simulink model "irep_force_control_m15"  (R2015a)
settings: Solver=ode3  StartTime=0.0  StopTime=inf  FixedStep=dt  RelTol=1e-3
InitFcn:
  | IREP_DEPENDENCY
  | init_omni
  | init_filters
  | init_invivo
  | init_telemanipulation
  | init_parker_xyz
  | init_magnetic_tracker
  | init_loadcell
  | init_scopes
  | init_homing
  | init_force_control
  | init_xpc_invivo_simu
undefined symbols (not defined in the file): ang_vel_scale, B_simu, beta, camera_home_voltage, counter_offset, dt, dt_trakstar, E_Y, encoder_counts, epsilon_robust_inverse, FS_LUT_TAU, FS_LUT_WE, gear_ratio, HomingFineEps, HomingRoughEps, HomingRoughVelocity, I1_primary, I1_secondary, I2_primary, I2_secondary, irep_parameters_left, irep_parameters_right, joystick_filter_coeffs, K_d, K_i, K_naive_inv, K_p, k_right, L1l, L1r, L2l, L2r, L_zeus, left_arm_home_voltage, left_x0_parallelogram, LeftArmHomingDirectionVector, LeftArmHomingIntGain, lin_vel_scale, LOADCELL_BIAS, LOADCELL_GAIN, max_conf_space_speed, N_joystick, N_pots, N_trakstar, OmegaMax, OmegaMin, orientation_epsilon, position_epsilon, pots_filter_coeffs, q_eps_backlash, quadrature_mode, r, right_arm_home_voltage, RightArmHomingDirectionVector, RightArmHomingIntGain, screw_pitch, statics_param, tau_compression_bias, tau_compression_gains, tau_neutral_deadband ... (+16)
libraries: slrtlib x39, simulink x23, xpcobsoletelib x23, xpcconteclib x23, xpcrtudplib x12, xpcmeasurementcomputinglib x6, dspswit3 x2, dspsigops x1
(part 2 of 7)

== system irep_force_control_m15/Joint Level PID Control in mm/Bus Creator ==
  In1 : Inport
  Bus Creator : BusCreator  Inputs=23
  Demux : Demux  Outputs=23
  Out1 : Outport
  wires:
  Demux/1 -> Bus Creator/1  "Righ arm - Overall Translational Movement"
  Demux/2 -> Bus Creator/2  "Right arm - Parallelogram Insert"
  Demux/3 -> Bus Creator/3  "Right arm - Parallelogram Deploy"
  Demux/4 -> Bus Creator/4  "Right arm - Proximal Segment X"
  Demux/5 -> Bus Creator/5  "Right arm - Proximal Segment Y"
  Demux/6 -> Bus Creator/6  "Right arm - Distal Segment X"
  Demux/7 -> Bus Creator/7  "Right arm - Distal Segment Y"
  Demux/8 -> Bus Creator/8  "Right arm - Wrist Joint"
  Demux/9 -> Bus Creator/9  "Right arm - Gripper Joint"
  Demux/10 -> Bus Creator/10  "Left arm - Overall Translational Movement"
  Demux/11 -> Bus Creator/11  "Left arm - Parallelogram Insert"
  Demux/12 -> Bus Creator/12  "Left arm - Parallelogram Deploy"
  Demux/13 -> Bus Creator/13  "Left arm - Proximal Segment X"
  Demux/14 -> Bus Creator/14  "Left arm - Proximal Segment Y"
  Demux/15 -> Bus Creator/15  "Left arm - Distal Segment X"
  Demux/16 -> Bus Creator/16  "Left arm - Distal Segment Y"
  Demux/17 -> Bus Creator/17  "Left arm - Wrist Joint"
  Demux/18 -> Bus Creator/18  "Left arm - Gripper Joint"
  Demux/19 -> Bus Creator/19  "Camera shell open"
  Demux/20 -> Bus Creator/20  "Camera Pan"
  Demux/21 -> Bus Creator/21  "Camera Tilt"
  Bus Creator/1 -> Out1/1
  In1/1 -> Demux/1
  Demux/22 -> Bus Creator/22  "Parker insertion stage"
  Demux/23 -> Bus Creator/23  "Parker rotary stage"

== system irep_force_control_m15/Joint Level PID Control in mm/Bus selector ==
  sensors : Inport
  Camera selector : Subsystem
  Left arm selector : Subsystem
  Mux : Mux
  RZ : Subsystem
  Right arm selector : Subsystem
  Out1 : Outport
  wires:
  Left arm selector/1(Out1) -> Mux/2
  Right arm selector/1(Out1) -> Mux/1
  Camera selector/1(Out1) -> Mux/3
  Mux/1 -> Out1/1
  sensors/1 -> Left arm selector/1(In1), Right arm selector/1(In1), Camera selector/1(In1), RZ/1(In1)
  RZ/1(Out1) -> Mux/4

== system irep_force_control_m15/Joint Level PID Control in mm/PID Compensator ==
  e : Inport
  Enable : EnablePort  StatesWhenEnabling=reset
  Add : Sum  Inputs=+++
  Discrete Derivative : simulink/Discrete/Discrete Derivative  gainval=1.0  ICPrevScaledInput=0.0  InputProcessing=Inherited  OutMin=[]  OutMax=[]  OutDataType=sfix(16)  OutScaling=2^-10  DoSatur=off
  Discrete-Time Integrator : DiscreteIntegrator  SampleTime=dt
  Integral Sat : Saturate  UpperLimit=5  LowerLimit=-5
  Kd : Gain  Gain=K_d  SampleTime=dt
  Ki : Gain  Gain=K_i  SampleTime=dt
  Kp : Gain  Gain=K_p  SampleTime=dt
  Saturation : Saturate  UpperLimit=10  LowerLimit=-10
  u : Outport  InitialOutput=zeros(23,1)
  wires:
  Discrete Derivative/1 -> Add/3
  Kd/1 -> Discrete Derivative/1
  Integral Sat/1 -> Add/2
  Discrete-Time Integrator/1 -> Integral Sat/1
  Saturation/1 -> u/1
  Add/1 -> Saturation/1
  Ki/1 -> Discrete-Time Integrator/1
  Kp/1 -> Add/1
  e/1 -> Ki/1, Kp/1, Kd/1

== system irep_force_control_m15/Scopes/Friction Estimation Data UDP ==
  note: ConfigSpace:
      | b0 [1x1]
      | b1 [2x1]
      | psi [4x1]
      | gamma [1x1]
  note: [9x1]
  note: [4x1]
  note: [6x1]
  note: [6x1]
  note: [6x1]
  note: [6x1]
  sensors : Inport
  ConfigComd : Inport  Port=2
  Clock : Inport  Port=3
  Enable : EnablePort
  Bus Selector1 : BusSelector  OutputSignals=Magnetic Sensors.s1,Magnetic Sensors.s2,Magnetic Sensors.s3,Magnetic Sensors.s4
  Bus Selector2 : BusSelector  OutputSignals=force_sensing.loadcell
  Bus Selector4 : BusSelector  OutputSignals=A/D signals.right arm pots
  Demux : Demux  Outputs=[1 6 1]
  Demux2 : Demux  Outputs=[9 1]
  Mux : Mux  Inputs=10
  Right arm joint def : Subsystem
  STOP : Constant  Value=0
  Terminator{,1..3} (4 alike) : Terminator
  wires:
  sensors/1 -> Right arm joint def/1(sensors), Bus Selector4/1, Bus Selector2/1, Bus Selector1/1
  Bus Selector2/1 -> Mux/3  "<loadcell>"
  Bus Selector1/1 -> Mux/4  "<s1>"
  Bus Selector1/2 -> Mux/5  "<s2>"
  Bus Selector1/3 -> Mux/6  "<s3>"
  Bus Selector1/4 -> Mux/7  "<s4>"
  Right arm joint def/1(right q_cur) -> Mux/1  "q_cur [9x1]"
  ConfigComd/1 -> Demux/1
  Demux/1 -> Terminator/1
  Demux/2 -> Mux/8  "b,psi [6x1]"
  Clock/1 -> Mux/9  "clock [1x1]"
  Mux/1 -> Terminator3/1
  STOP/1 -> Mux/10
  Demux/3 -> Terminator1/1
  Bus Selector4/1 -> Demux2/1  "<right arm pots>"
  Demux2/1 -> Mux/2
  Demux2/2 -> Terminator2/1

== system irep_force_control_m15/Scopes/Left arm joint def ==
  In1 : Inport
  Bus Selector5 : BusSelector  OutputSignals=q.Left arm - overall translational movement,q.Left arm - parallelogram insert joint,q.Left arm - parallelogram deployment joint,q.Left arm - proximal segment - bending in X,q.Left arm - proximal segment - bending in Y,q.Left arm - distal segment - bending in x,q.Left arm - distal segment - bending in y,q.Left arm - wrist,q.Left arm - gripper joint
  Mux5 : Mux  Inputs=9
  Out1 : Outport
  wires:
  Bus Selector5/1 -> Mux5/1  "<Left arm - overall translational movement>"
  Bus Selector5/2 -> Mux5/2  "<Left arm - parallelogram insert joint>"
  Bus Selector5/3 -> Mux5/3  "<Left arm - parallelogram deployment joint>"
  Bus Selector5/4 -> Mux5/4  "<Left arm - proximal segment - bending in X>"
  Bus Selector5/5 -> Mux5/5  "<Left arm - proximal segment - bending in Y>"
  Bus Selector5/6 -> Mux5/6  "<Left arm - distal segment - bending in x>"
  Bus Selector5/7 -> Mux5/7  "<Left arm - distal segment - bending in y>"
  Bus Selector5/8 -> Mux5/8  "<Left arm - wrist>"
  Bus Selector5/9 -> Mux5/9  "<Left arm - gripper joint>"
  In1/1 -> Bus Selector5/1
  Mux5/1 -> Out1/1

== system irep_force_control_m15/Scopes/Magnetic Sensor Scopes ==
  In1 : Inport
  Bus Selector4 : BusSelector  OutputSignals=Magnetic Sensors.s1
  Bus Selector5 : BusSelector  OutputSignals=Magnetic Sensors.s2
  Bus Selector6 : BusSelector  OutputSignals=Magnetic Sensors.s3
  Bus Selector7 : BusSelector  OutputSignals=Magnetic Sensors.s4
  Scope M sensor 1 : slrtlib/Displays and Logging/Scope   scopeno=22  scopetype=Host  autostart=on  viewmode=Numerical  formatstr=scope_format_Msensor_1  grid=on  ylimits=[0,0]  nosamples=50  noprepostsamples=0  interleave=1  triggermode=FreeRun  triggersignal=1  trigsignalfromport=off  triggerlevel=0.0  triggerslope=Either  triggerscope=1  triggersample=0  filename=data.dat  mode=Lazy  writesize=512  autorestart=off  dynamicfilemode=off  maxwritefilesize=512*1024^2
  Scope M sensor 2 : slrtlib/Displays and Logging/Scope   scopeno=23  scopetype=Host  autostart=off  viewmode=Numerical  formatstr=scope_format_Msensor_2  grid=on  ylimits=[0,0]  nosamples=50  noprepostsamples=0  interleave=1  triggermode=FreeRun  triggersignal=1  trigsignalfromport=off  triggerlevel=0.0  triggerslope=Either  triggerscope=1  triggersample=0  filename=data.dat  mode=Lazy  writesize=512  autorestart=off  dynamicfilemode=off  maxwritefilesize=512*1024^2
  "Scope M sensor 3 " : slrtlib/Displays and Logging/Scope   scopeno=30  scopetype=Host  autostart=on  viewmode=Numerical  formatstr=scope_format_Msensor_3  grid=on  ylimits=[0,0]  nosamples=50  noprepostsamples=0  interleave=1  triggermode=FreeRun  triggersignal=1  trigsignalfromport=off  triggerlevel=0.0  triggerslope=Either  triggerscope=1  triggersample=0  filename=data.dat  mode=Lazy  writesize=512  autorestart=off  dynamicfilemode=off  maxwritefilesize=512*1024^2
  Scope M sensor 4 : slrtlib/Displays and Logging/Scope   scopeno=31  scopetype=Host  autostart=on  viewmode=Numerical  formatstr=scope_format_Msensor_4  grid=on  ylimits=[0,0]  nosamples=50  noprepostsamples=0  interleave=1  triggermode=FreeRun  triggersignal=1  trigsignalfromport=off  triggerlevel=0.0  triggerslope=Either  triggerscope=1  triggersample=0  filename=data.dat  mode=Lazy  writesize=512  autorestart=off  dynamicfilemode=off  maxwritefilesize=512*1024^2
  wires:
  Bus Selector4/1 -> Scope M sensor 1/1  "<s1>"
  Bus Selector5/1 -> Scope M sensor 2/1  "<s2>"
  Bus Selector6/1 -> "Scope M sensor 3 "/1  "<s3>"
  Bus Selector7/1 -> Scope M sensor 4/1  "<s4>"
  In1/1 -> Bus Selector6/1, Bus Selector7/1, Bus Selector5/1, Bus Selector4/1

== system irep_force_control_m15/Scopes/Other_scope ==
  In1 : Inport
  Bus Selector2 : BusSelector  OutputSignals=A/D signals.right arm pots,A/D signals.left arm pots,q.Parker insertion stage,q.Parker rotary stage,q.Camera shell open,q.Camera Pan,q.Camera Tilt,foot switches,Pots_Connect
  Camera : slrtlib/Displays and Logging/Scope   scopeno=6  scopetype=Host  autostart=on  viewmode=Numerical  formatstr='Camera: %3.3f'  grid=on  ylimits=[0,0]  nosamples=10  noprepostsamples=0  interleave=1  triggermode=FreeRun  triggersignal=1  trigsignalfromport=off  triggerlevel=0.0  triggerslope=Either  triggerscope=1  triggersample=0  filename=weights1.dat  mode=Lazy  writesize=512  autorestart=off  dynamicfilemode=off  maxwritefilesize=512*1024^2
  Digital Input : slrtlib/Displays and Logging/Scope   scopeno=2  scopetype=Host  autostart=on  viewmode=Numerical  formatstr=scope_format_digital_input  grid=on  ylimits=[0,0]  nosamples=10  noprepostsamples=0  interleave=1  triggermode=FreeRun  triggersignal=1  trigsignalfromport=off  triggerlevel=0.0  triggerslope=Either  triggerscope=1  triggersample=0  filename=weights1.dat  mode=Lazy  writesize=512  autorestart=off  dynamicfilemode=off  maxwritefilesize=512*1024^2
  Left Arm Pots : slrtlib/Displays and Logging/Scope   scopeno=7  scopetype=Target  autostart=on  viewmode=Numerical  formatstr=scope_format_left_pot  grid=on  ylimits=[0,0]  nosamples=10  noprepostsamples=0  interleave=1  triggermode=FreeRun  triggersignal=1  trigsignalfromport=off  triggerlevel=0.0  triggerslope=Either  triggerscope=1  triggersample=0  filename=weights1.dat  mode=Lazy  writesize=512  autorestart=off  dynamicfilemode=off  maxwritefilesize=512*1024^2
  Mux2 : Mux  Inputs=2
  Mux3 : Mux  Inputs=3
  Mux4 : Mux  Inputs=2
  Parker Feedback : slrtlib/Displays and Logging/Scope   scopeno=4  scopetype=Host  autostart=on  viewmode=Numerical  formatstr=scope_format_parker_cur  grid=on  ylimits=[0,0]  nosamples=10  noprepostsamples=0  interleave=1  triggermode=FreeRun  triggersignal=1  trigsignalfromport=off  triggerlevel=0.0  triggerslope=Either  triggerscope=1  triggersample=0  filename=weights1.dat  mode=Lazy  writesize=512  autorestart=off  dynamicfilemode=off  maxwritefilesize=512*1024^2
  Right Arm Pots : slrtlib/Displays and Logging/Scope   scopeno=8  scopetype=Target  autostart=on  viewmode=Numerical  formatstr=scope_format_right_pot  grid=on  ylimits=[0,0]  nosamples=10  noprepostsamples=0  interleave=1  triggermode=FreeRun  triggersignal=1  trigsignalfromport=off  triggerlevel=0.0  triggerslope=Either  triggerscope=1  triggersample=0  filename=weights1.dat  mode=Lazy  writesize=512  autorestart=off  dynamicfilemode=off  maxwritefilesize=512*1024^2
  wires:
  Bus Selector2/1 -> Right Arm Pots/1  "<right arm pots>"
  Bus Selector2/2 -> Left Arm Pots/1  "<left arm pots>"
  Bus Selector2/3 -> Mux2/1  "<Parker insertion stage>"
  Bus Selector2/4 -> Mux2/2  "<Parker rotary stage>"
  Mux2/1 -> Parker Feedback/1
  Mux3/1 -> Camera/1
  Bus Selector2/5 -> Mux3/1  "<Camera shell open>"
  Bus Selector2/6 -> Mux3/2  "<Camera Pan>"
  Bus Selector2/7 -> Mux3/3  "<Camera Tilt>"
  Bus Selector2/8 -> Mux4/1  "<foot switches>"
  Bus Selector2/9 -> Mux4/2  "<Pots_Connect>"
  Mux4/1 -> Digital Input/1
  In1/1 -> Bus Selector2/1

== system irep_force_control_m15/Scopes/Right arm joint def ==
  In1 : Inport
  Bus Selector4 : BusSelector  OutputSignals=q.Right arm - overall translational movement,q.Right arm - parallelogram insert joint,q.Right arm - parallelogram deployment joint,q.Right arm - Proximal segment - bending in X,q.Righ arm - Proximal segment - bending in Y,q.Right arm - distal segment - bending in X,q.Right arm - distal segment - bending in Y,q.Right arm - wrist,q.Right arm - Gripper Joint
  Mux1 : Mux  Inputs=9
  Out1 : Outport
  wires:
  Bus Selector4/1 -> Mux1/1  "<Right arm - overall translational movement>"
  Bus Selector4/2 -> Mux1/2  "<Right arm - parallelogram insert joint>"
  Bus Selector4/3 -> Mux1/3  "<Right arm - parallelogram deployment joint>"
  Bus Selector4/4 -> Mux1/4  "<Right arm - Proximal segment - bending in X>"
  Bus Selector4/5 -> Mux1/5  "<Righ arm - Proximal segment - bending in Y>"
  Bus Selector4/6 -> Mux1/6  "<Right arm - distal segment - bending in X>"
  Bus Selector4/7 -> Mux1/7  "<Right arm - distal segment - bending in Y>"
  Bus Selector4/8 -> Mux1/8  "<Right arm - wrist>"
  Bus Selector4/9 -> Mux1/9  "<Right arm - Gripper Joint>"
  In1/1 -> Bus Selector4/1
  Mux1/1 -> Out1/1

== system irep_force_control_m15/Scopes/left ==
  In1 : Inport
  Bus Selector : BusSelector  OutputSignals=Left arm - Proximal Segment Y,Left arm - Gripper Joint,Left arm - Proximal Segment X,Left arm - Distal Segment X,Left arm - Wrist Joint,Left arm - Distal Segment Y,Left arm - Parallelogram Deploy,Left arm - Parallelogram Insert,Left arm - Overall Translational Movement
  Gain{1..4} (4 alike) : Gain  Gain=-1
  Mux : Mux  Inputs=9
  Out1 : Outport
  wires:
  Bus Selector/1 -> Gain1/1  "<Left arm - Proximal Segment Y>"
  Bus Selector/2 -> Mux/2  "<Left arm - Gripper Joint>"
  Bus Selector/4 -> Mux/4  "<Left arm - Distal Segment X>"
  Bus Selector/5 -> Mux/5  "<Left arm - Wrist Joint>"
  Bus Selector/6 -> Gain2/1  "<Left arm - Distal Segment Y>"
  Bus Selector/7 -> Gain3/1  "<Left arm - Parallelogram Deploy>"
  Bus Selector/8 -> Gain4/1  "<Left arm - Parallelogram Insert>"
  In1/1 -> Bus Selector/1
  Mux/1 -> Out1/1
  Bus Selector/3 -> Mux/3  "<Left arm - Proximal Segment X>"
  Gain1/1 -> Mux/1
  Gain2/1 -> Mux/6
  Gain3/1 -> Mux/7
  Gain4/1 -> Mux/8
  Bus Selector/9 -> Mux/9  "<Left arm - Overall Translational Movement>"

== system irep_force_control_m15/Scopes/parker ==
  In1 : Inport
  Bus Selector : BusSelector  OutputSignals=Parker insertion stage,Parker rotary stage
  Gain1 : Gain  Gain=-1
  Gain2 : Gain  Gain=-1
  Mux : Mux  Inputs=2
  Out1 : Outport
  wires:
  Bus Selector/1 -> Gain1/1  "<Parker insertion stage>"
  Bus Selector/2 -> Gain2/1  "<Parker rotary stage>"
  In1/1 -> Bus Selector/1
  Mux/1 -> Out1/1
  Gain1/1 -> Mux/1
  Gain2/1 -> Mux/2

== system irep_force_control_m15/Scopes/right ==
  In1 : Inport
  Bus Selector : BusSelector  OutputSignals=Right arm - Proximal Segment Y,Right arm - Gripper Joint,Right arm - Proximal Segment X,Right arm - Distal Segment X,Right arm - Wrist Joint,Right arm - Distal Segment Y,Right arm - Parallelogram Deploy,Right arm - Parallelogram Insert,Righ arm - Overall Translational Movement
  Mux : Mux  Inputs=9
  Out1 : Outport
  wires:
  In1/1 -> Bus Selector/1
  Mux/1 -> Out1/1
  Bus Selector/3 -> Mux/3  "<Right arm - Proximal Segment X>"
  Bus Selector/4 -> Mux/4  "<Right arm - Distal Segment X>"
  Bus Selector/5 -> Mux/5  "<Right arm - Wrist Joint>"
  Bus Selector/6 -> Mux/6  "<Right arm - Distal Segment Y>"
  Bus Selector/8 -> Mux/8  "<Right arm - Parallelogram Insert>"
  Bus Selector/2 -> Mux/2  "<Right arm - Gripper Joint>"
  Bus Selector/1 -> Mux/1  "<Right arm - Proximal Segment Y>"
  Bus Selector/7 -> Mux/7  "<Right arm - Parallelogram Deploy>"
  Bus Selector/9 -> Mux/9  "<Righ arm - Overall Translational Movement>"

== system irep_force_control_m15/Scopes/select force ==
  wrench est : Inport
  Bus Selector4 : BusSelector  OutputSignals=Ws_right,Ws_uncomp,We_right_seg1,Ws_bias
  Demux{,1..3} (4 alike) : Demux  Outputs=[3,3]
  Mux : Mux  Inputs=3
  Terminator{,1..4} (5 alike) : Terminator
  Force : Outport
  wires:
  Bus Selector4/1 -> Demux/1  "<Ws_right>"
  Bus Selector4/3 -> Demux1/1  "<We_right_seg1>"
  Demux/2 -> Terminator/1  "Torque"
  Demux1/2 -> Terminator1/1  "Torque"
  Demux/1 -> Mux/1  "Force"
  Mux/1 -> Force/1
  wrench est/1 -> Bus Selector4/1
  Demux1/1 -> Terminator2/1  "Force"
  Bus Selector4/2 -> Demux2/1  "<Ws_uncomp>"
  Demux2/2 -> Terminator3/1
  Demux2/1 -> Mux/2
  Bus Selector4/4 -> Demux3/1  "<Ws_bias>"
  Demux3/2 -> Terminator4/1
  Demux3/1 -> Mux/3

== system irep_force_control_m15/Trajectory Planner/Camera ==
  vision : Inport
  sensors : Inport  Port=2
  Enable : EnablePort
  Enable Homing : Constant  Value=0  SampleTime=dt
  Enable Joint Space : Constant  Value=0  SampleTime=dt
  Enable Joystick : Constant  Value=0  SampleTime=dt
  Enable Tool Tracking : Constant  Value=0  SampleTime=dt
  Homing Procedure : Subsystem  TreatAsAtomicUnit=on
  Joint Space : Subsystem  TreatAsAtomicUnit=on
  Joystick Control for Cam : Subsystem  TreatAsAtomicUnit=on
  Merge : Merge  Inputs=4  InitialOutput=zeros(3,1)
  Saturation : Saturate  UpperLimit=[5 1.6 1.5]  LowerLimit=[-5 -1.6 -1.5]
  Tool Tracking : Subsystem  TreatAsAtomicUnit=on
  q des camera : Outport  InitialOutput=zeros(3,1)
  wires:
  Enable Tool Tracking/1 -> Tool Tracking/Enable
  Merge/1 -> Saturation/1
  vision/1 -> Tool Tracking/1(tool XY)
  Enable Joint Space/1 -> Joint Space/Enable
  sensors/1 -> Joystick Control for Cam/1(sensors), Homing Procedure/1(sensors)
  Enable Joystick/1 -> Joystick Control for Cam/Enable
  Homing Procedure/1(q des) -> Merge/1
  Joint Space/1(Out1) -> Merge/2
  Tool Tracking/1(q des) -> Merge/3
  Joystick Control for Cam/1(q des) -> Merge/4
  Enable Homing/1 -> Homing Procedure/Enable
  Saturation/1 -> q des camera/1

== system irep_force_control_m15/Trajectory Planner/Delay_test ==
  Delay_test : xpcrtudplib/Legacy UDP/Send   ipAddress=192.168.1.64  ipPort=10031  localPort=-1  vblLen=off  sampletime=0.01
  Digital Clock : DigitalClock  SampleTime=dt
  Pack1 : xpcobsoletelib/Utilities/Pack   datatypes={'double'}  byteAlign=1
  Receive : xpcrtudplib/Legacy UDP/Receive   ipAddress=0.0.0.0  ipPort=10030  width=8  vblLen=on  sampletime=0.01
  "Scope (xPC) " : slrtlib/Displays and Logging/Scope   scopeno=25  scopetype=Host  autostart=on  viewmode=Numerical  formatstr='Delay:%15.6f'  grid=on  ylimits=[0,0]  nosamples=250  noprepostsamples=0  interleave=1  triggermode=FreeRun  triggersignal=1  trigsignalfromport=off  triggerlevel=0.0  triggerslope=Either  triggerscope=1  triggersample=0  filename=data.dat  mode=Lazy  writesize=512  autorestart=off  dynamicfilemode=off  maxwritefilesize=512*1024^2
  Sum : Sum  Inputs=|+-
  Terminator : Terminator
  Unpack : xpcobsoletelib/Utilities/Unpack   dimensions={1}  datatypes={'double'}  byteAlign=1
  wires:
  Digital Clock/1 -> Pack1/1, Sum/1
  Pack1/1 -> Delay_test/1
  Receive/2 -> Terminator/1
  Receive/1 -> Unpack/1
  Unpack/1 -> Sum/2
  Sum/1 -> "Scope (xPC) "/1

== system irep_force_control_m15/Trajectory Planner/Left Arm ==
  note: IREP Left Arm Trajectory Planner - v 0.6 - © COPYRIGHT 2011 Andrea Bajo, Nabil Simaan
  Master : Inport
  sensors : Inport  Port=2
  Enable : EnablePort
  Enable High Level : Constant  Value=0  SampleTime=dt
  Enable Low Level : Constant  Value=0  SampleTime=dt
  High Level : Subsystem  TreatAsAtomicUnit=on
  Low Level : Subsystem  TreatAsAtomicUnit=on
  Merge1 : Merge  InitialOutput=zeros(9,1)
  q left arm : Outport  InitialOutput=zeros(9,1)
  conf space : Outport  Port=2
  b0 dot left : Outport  Port=3
  TASK_EN : Outport  Port=4
  current_pose : Outport  Port=5
  wires:
  Enable Low Level/1 -> Low Level/Enable
  Low Level/1(q des) -> Merge1/1
  Enable High Level/1 -> High Level/Enable
  High Level/1(q des) -> Merge1/2
  sensors/1 -> Low Level/1(sensors), High Level/2(sensors)
  Master/1 -> High Level/1(Master)
  Merge1/1 -> q left arm/1
  High Level/2(conf space) -> conf space/1
  High Level/3(b0_dot_left) -> b0 dot left/1
  High Level/4(TASK_EN) -> TASK_EN/1
  High Level/5(current_pose) -> current_pose/1

== system irep_force_control_m15/Trajectory Planner/RZ ==
  trajectory : Inport
  sensors : Inport  Port=2
  Enable : EnablePort
  Add : Sum
  Arm selector : MATLAB Function  TreatAsAtomicUnit=on
  Bus Selector1 : BusSelector  OutputSignals=right arm.b0 dot right,left arm.b0 dot left
  Discrete-Time Integrator : DiscreteIntegrator  InitialCondition=[0;0]  SampleTime=dt  LimitOutput=on  UpperSaturationLimit=[200;pi/2]  LowerSaturationLimit=[-100;0]
  Enable Joint Space : Constant  Value=0  SampleTime=dt
  Joystick Control for RZ : Subsystem  TreatAsAtomicUnit=on
  Subsystem : Subsystem
  Parker : Outport  InitialOutput=zeros(2,1)
  wires:
  sensors/1 -> Joystick Control for RZ/1(sensors)
  Joystick Control for RZ/1(q des) -> Subsystem/1(In1)
  Enable Joint Space/1 -> Joystick Control for RZ/Enable
  Add/1 -> Discrete-Time Integrator/1
  Subsystem/1(Out1) -> Add/2
  Arm selector/1(b0dot) -> Add/1
  Discrete-Time Integrator/1 -> Parker/1
  trajectory/1 -> Bus Selector1/1
  Bus Selector1/1 -> Arm selector/1(right_b0_dot)  "<b0 dot right>"
  Bus Selector1/2 -> Arm selector/2(left_b0_dot)  "<b0 dot left>"

== system irep_force_control_m15/Trajectory Planner/Right Arm ==
  note: IREP Right Arm Trajectory Planner - v 1.0 - © COPYRIGHT 2011 Andrea Bajo, Nabil Simaan
  Master : Inport
  sensors : Inport  Port=2
  Enable : EnablePort
  Enable High Level : Constant  Value=0  SampleTime=dt
  Enable Low Level : Constant  Value=0  SampleTime=dt
  High Level : Subsystem  TreatAsAtomicUnit=on
  Low Level : Subsystem  TreatAsAtomicUnit=on
  Merge1 : Merge  InitialOutput=zeros(9,1)
  conf space : Outport  PortDimensions=8
  q right arm : Outport  Port=2  InitialOutput=zeros(9,1)
  b0 dot right : Outport  Port=3
  TASK_EN : Outport  Port=4
  current_pose : Outport  Port=5
  q dot sgn : Outport  Port=6
  wires:
  Enable Low Level/1 -> Low Level/Enable
  Low Level/1(q des) -> Merge1/1
  Enable High Level/1 -> High Level/Enable
  High Level/1(q des) -> Merge1/2
  sensors/1 -> Low Level/1(sensors), High Level/2(sensors)
  Master/1 -> High Level/1(Master)
  High Level/2(conf space) -> conf space/1
  High Level/3(b0 dot) -> b0 dot right/1
  High Level/4(TASK_EN) -> TASK_EN/1
  Merge1/1 -> q right arm/1
  High Level/5(current_pose) -> current_pose/1
  High Level/6(q dot sgn) -> q dot sgn/1

== system irep_force_control_m15/Trajectory Planner/Signals packing ==
  irep : Inport
  parker : Inport  Port=2
  Bus Creator : BusCreator
  Bus Selector : BusSelector  OutputSignals=right arm.q des right,left arm.q des left,camera q
  system : Outport
  wires:
  Bus Selector/1 -> Bus Creator/1  "<q des right>"
  Bus Selector/2 -> Bus Creator/2  "<q des left>"
  Bus Selector/3 -> Bus Creator/3  "<camera q>"
  irep/1 -> Bus Selector/1
  Bus Creator/1 -> system/1
  parker/1 -> Bus Creator/4

== system irep_force_control_m15/Trajectory Planner/UDP_SendTo_MTM ==
  Traj : Inport
  Right_MTM : Inport  Port=2
  Left_MTM : Inport  Port=3
  Right_Wrench : Inport  Port=4
  Left_UDP : Subsystem
  Right_UDP : Subsystem
  wires:
  Traj/1 -> Right_UDP/1(traj), Left_UDP/1(traj)
  Right_MTM/1 -> Right_UDP/2(MTM)
  Left_MTM/1 -> Left_UDP/2(MTM)
  Right_Wrench/1 -> Right_UDP/3(Wrench)

== system irep_force_control_m15/Wrench Estimation/Wrench Compensation ==
  note: Compensation Mode
  note: Compensation using lookup tables
  Ws : Inport
  q_dot_sign : Inport  Port=2
  psi : Inport  Port=3
  Compare To Constant1 : simulink/Logic and Bit Operations/Compare To Constant  relop===  const=1  OutDataTypeStr=boolean
  Constant : Constant  Value=zeros(12,1)
  Multiport Switch : MultiPortSwitch  DataPortOrder=Specify indices  DataPortIndices={1,0}
  Sum : Sum  Inputs=+-|
  wrench comp mode : Constant  Value=0
  wrench sensing compensation LUT : Subsystem
  Ws_comp : Outport
  Ws_bias : Outport  Port=2
  wires:
  [mode] -> Multiport Switch/1
  wrench comp mode/1 -> [mode]
  Multiport Switch/1 -> Ws_bias/1, Sum/2
  [mode] -> Compare To Constant1/1
  Compare To Constant1/1 -> wrench sensing compensation LUT/Enable
  q_dot_sign/1 -> wrench sensing compensation LUT/1(q_dot_sign)
  psi/1 -> wrench sensing compensation LUT/2(psi)
  wrench sensing compensation LUT/1(ws_bias) -> Multiport Switch/2
  Ws/1 -> Sum/1
  Sum/1 -> Ws_comp/1
  Constant/1 -> Multiport Switch/3

== system irep_force_control_m15/Wrench Estimation/Wrench Est Right Arm ==
  note: Ws - the estimated wrench at the tip of the robot
      | We_seg1 - the estimated wrench at the end of the 1st segment
      | tau_comp - the compensated tau
  tau : Inport
  psi : Inport  Port=2
  Constant : Constant  Value=r
  Constant1 : Constant  Value=[1 0 0]
  Constant2 : Constant  Value=[0 1 0]
  Constant3 : Constant
  Constant4 : Constant
  Constant5 : Constant  Value=0
  Mux : Mux  Inputs=2
  Sample and Hold : dspsigops/Sample and Hold  trig=Rising edge  initCond=0  latchinput=off
  Sum : Sum  Inputs=|+-
  compute wrench est : MATLAB Function  TreatAsAtomicUnit=on
  reset : Constant  Value=0
  robot kin param : Constant  Value=irep_parameters_right
  robot statics param : Constant  Value=statics_param
  sel param : Subsystem
  Ws : Outport
  wires:
  Constant/1 -> compute wrench est/8(r)
  Constant1/1 -> compute wrench est/3(n_t)
  Constant2/1 -> compute wrench est/4(n_n)
  Constant3/1 -> compute wrench est/5(c_t)
  Constant4/1 -> compute wrench est/6(c_n)
  robot kin param/1 -> sel param/1(In)
  sel param/1(L) -> compute wrench est/7(L)
  robot statics param/1 -> compute wrench est/9(statics_param)
  Constant5/1 -> compute wrench est/10(probe_offset)
  psi/1 -> compute wrench est/2(Psi)
  tau/1 -> compute wrench est/1(tau_curr)
  reset/1 -> Sample and Hold/Trigger
  Mux/1 -> Sum/1, Sample and Hold/1
  Sample and Hold/1 -> Sum/2
  compute wrench est/1(Ws) -> Mux/1
  compute wrench est/2(W_seg1) -> Mux/2
  Sum/1 -> Ws/1

== system irep_force_control_m15/Wrench Estimation/combine psi ==
  note: Combining measured psi and commanded psi
      | measured psi has a good estimate of theta
      | but very poor estimate of delta
  psi_d : Inport
  psi_m : Inport  Port=2
  Demux : Demux  Outputs=[4,1]
  Sum : Sum  Inputs=|++
  Terminator : Terminator
  select desired : Gain  Gain=[1,1,1,1]
  select measured : Gain  Gain=[0,0,0,0]
  psi : Outport
  wires:
  psi_m/1 -> select measured/1
  Sum/1 -> psi/1
  Demux/2 -> Terminator/1
  Demux/1 -> select desired/1
  select measured/1 -> Sum/1
  select desired/1 -> Sum/2
  psi_d/1 -> Demux/1

== system irep_force_control_m15/Wrench Estimation/q_cur to q_bb ==
  q_cur : Inport
  Bus Selector1 : BusSelector  OutputSignals=q.Right arm - Proximal segment - bending in X,q.Righ arm - Proximal segment - bending in Y,q.Right arm - distal segment - bending in X,q.Right arm - distal segment - bending in Y
  Gain{,1..3} (4 alike) : Gain  Gain=-1
  Mux1 : Mux  Inputs=8
  q_bb : Outport
  wires:
  q_cur/1 -> Bus Selector1/1
  Mux1/1 -> q_bb/1
  Bus Selector1/1 -> Mux1/1, Gain/1  "<Right arm - Proximal segment - bending in X>"
  Bus Selector1/2 -> Mux1/2, Gain1/1  "<Righ arm - Proximal segment - bending in Y>"
  Bus Selector1/3 -> Mux1/5, Gain2/1  "<Right arm - distal segment - bending in X>"
  Bus Selector1/4 -> Mux1/6, Gain3/1  "<Right arm - distal segment - bending in Y>"
  Gain/1 -> Mux1/3
  Gain1/1 -> Mux1/4
  Gain2/1 -> Mux1/7
  Gain3/1 -> Mux1/8

== system irep_force_control_m15/Wrench Estimation/signal packing ==
  note: Ws_right - the estimated wrench at the tip of the robot
      | We_right_seg1 - the estimated wrench at the end of the 1st segment
      | tau_comp - the compensated tau
  tau_comp : Inport
  Ws : Inport  Port=2
  Ws_uncomp : Inport  Port=3
  Ws_bias : Inport  Port=4
  Bus Creator : BusCreator  Inputs=5
  Demux : Demux  Outputs=[6,6]
  Demux1 : Demux  Outputs=[6,6]
  Demux2 : Demux  Outputs=[6,6]
  Terminator : Terminator
  Terminator1 : Terminator
  wrench_est : Outport
  wires:
  Ws/1 -> Demux/1
  Demux/1 -> Bus Creator/2  "Ws_right"
  tau_comp/1 -> Bus Creator/1  "tau_comp"
  Demux/2 -> Bus Creator/3  "We_right_seg1"
  Bus Creator/1 -> wrench_est/1  "wrench_est"
  Ws_uncomp/1 -> Demux1/1
  Demux1/2 -> Terminator/1
  Demux1/1 -> Bus Creator/4  "Ws_uncomp"
  Ws_bias/1 -> Demux2/1
  Demux2/2 -> Terminator1/1
  Demux2/1 -> Bus Creator/5  "Ws_bias"

== system irep_force_control_m15/Wrench Estimation/tau sensing compensation ==
  note: Compensation using gain model
  note: Compensation using lookup tables
  note: Compensation Mode
  q_bb : Inport
  tau_measured : Inport  Port=2
  q_dot_sign : Inport  Port=3
  psi : Inport  Port=4
  Compare To Constant : simulink/Logic and Bit Operations/Compare To Constant  relop===  const=1  OutDataTypeStr=boolean
  Compare To Constant1 : simulink/Logic and Bit Operations/Compare To Constant  relop===  const=2  OutDataTypeStr=boolean
  Multiport Switch : MultiPortSwitch  DataPortOrder=Specify indices  DataPortIndices={1,2,0}
  tau comp mode : Constant  Value=0
  tau sensing compensation LUT : Subsystem
  tau sensing compensation gain model : Subsystem
  tau_comp : Outport
  wires:
  tau_measured/1 -> tau sensing compensation LUT/1(tau_measured), Multiport Switch/4, tau sensing compensation gain model/2(tau_sensed)
  q_bb/1 -> tau sensing compensation gain model/1(q_bb)
  tau comp mode/1 -> [mode]
  [mode] -> Compare To Constant/1
  Compare To Constant/1 -> tau sensing compensation gain model/Enable
  [mode] -> Compare To Constant1/1
  Compare To Constant1/1 -> tau sensing compensation LUT/Enable
  q_dot_sign/1 -> tau sensing compensation LUT/2(q_dot_sign)
  psi/1 -> tau sensing compensation LUT/3(psi)
  Multiport Switch/1 -> tau_comp/1
  tau sensing compensation gain model/1(tau_comp) -> Multiport Switch/2
  tau sensing compensation LUT/1(tau_comp) -> Multiport Switch/3
  [mode] -> Multiport Switch/1

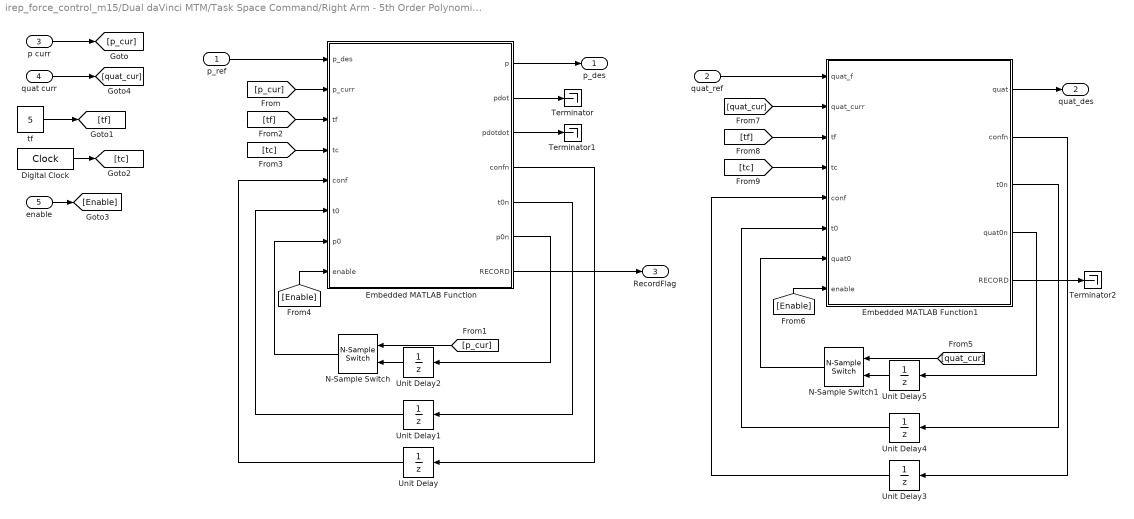
== system irep_force_control_m15/Dual daVinci MTM/Task Space Command/Right Arm - 5th Order Polynomial and Slerp ==
  p_ref : Inport
  quat_ref : Inport  Port=2
  p curr : Inport  Port=3
  quat curr : Inport  Port=4
  enable : Inport  Port=5
  Digital Clock : DigitalClock  SampleTime=dt
  Embedded MATLAB Function : MATLAB Function  TreatAsAtomicUnit=on
  Embedded MATLAB Function1 : MATLAB Function  TreatAsAtomicUnit=on
  N-Sample Switch : dspswit3/N-Sample Switch  N=1  reset=off  TriggerType=Rising edge  Ts=dt
  N-Sample Switch1 : dspswit3/N-Sample Switch  N=1  reset=off  TriggerType=Rising edge  Ts=dt
  Terminator : Terminator
  Terminator1 : Terminator
  Terminator2 : Terminator
  Unit Delay{,1..4} (5 alike) : UnitDelay  SampleTime=dt
  Unit Delay5 : UnitDelay  InitialCondition=[1;0;0;0]  SampleTime=dt
  tf : Constant  Value=5  SampleTime=dt
  p_des : Outport
  quat_des : Outport  Port=2
  RecordFlag : Outport  Port=3
  wires:
  Embedded MATLAB Function/4(confn) -> Unit Delay/1
  Unit Delay/1 -> Embedded MATLAB Function/5(conf)
  Embedded MATLAB Function/5(t0n) -> Unit Delay1/1
  Embedded MATLAB Function/6(p0n) -> Unit Delay2/1
  Unit Delay1/1 -> Embedded MATLAB Function/6(t0)
  p_ref/1 -> Embedded MATLAB Function/1(p_des)
  Embedded MATLAB Function/2(pdot) -> Terminator/1
  Embedded MATLAB Function/3(pdotdot) -> Terminator1/1
  N-Sample Switch/1 -> Embedded MATLAB Function/7(p0)
  Unit Delay2/1 -> N-Sample Switch/2
  p curr/1 -> [p_cur]
  [p_cur] -> Embedded MATLAB Function/2(p_curr)
  [p_cur] -> N-Sample Switch/1
  Embedded MATLAB Function/7(RECORD) -> RecordFlag/1
  Embedded MATLAB Function/1(p) -> p_des/1
  tf/1 -> [tf]
  Digital Clock/1 -> [tc]
  [tf] -> Embedded MATLAB Function/3(tf)
  [tc] -> Embedded MATLAB Function/4(tc)
  enable/1 -> [Enable]
  [Enable] -> Embedded MATLAB Function/8(enable)
  quat_ref/1 -> Embedded MATLAB Function1/1(quat_f)
  quat curr/1 -> [quat_cur]
  Embedded MATLAB Function1/3(t0n) -> Unit Delay4/1
  Embedded MATLAB Function1/4(quat0n) -> Unit Delay5/1
  Unit Delay4/1 -> Embedded MATLAB Function1/6(t0)
  N-Sample Switch1/1 -> Embedded MATLAB Function1/7(quat0)
  Unit Delay5/1 -> N-Sample Switch1/2
  [quat_cur] -> N-Sample Switch1/1
  Embedded MATLAB Function1/2(confn) -> Unit Delay3/1
  Unit Delay3/1 -> Embedded MATLAB Function1/5(conf)
  [Enable] -> Embedded MATLAB Function1/8(enable)
  [quat_cur] -> Embedded MATLAB Function1/2(quat_curr)
  [tf] -> Embedded MATLAB Function1/3(tf)
  [tc] -> Embedded MATLAB Function1/4(tc)
  Embedded MATLAB Function1/1(quat) -> quat_des/1
  Embedded MATLAB Function1/5(RECORD) -> Terminator2/1

== system irep_force_control_m15/Dual daVinci MTM/scopes/to file ==
  right : Inport
  left : Inport  Port=2
  Enable : EnablePort
  Joint Space Info File : slrtlib/Displays and Logging/Scope   scopeno=24  scopetype=File  autostart=on  viewmode=Numerical  formatstr="'tau: %8.3f,     %8.3f,     %8.3f,     %8.3f,     %8.3f,     %8.3f'"  grid=on  ylimits=[0,0]  nosamples=100000  noprepostsamples=0  interleave=1  triggermode=FreeRun  triggersignal=1  trigsignalfromport=off  triggerlevel=0.0  triggerslope=Either  triggerscope=1  triggersample=0  filename=MTMR.dat  mode=Lazy  writesize=512  autorestart=off  dynamicfilemode=off  maxwritefilesize=512*1024^2
  Terminator : Terminator
  wires:
  right/1 -> Joint Space Info File/1
  left/1 -> Terminator/1

== system irep_force_control_m15/In-Vivo System/CONTEC CARDS/Level 1 ==
  note: Contec
      | CNT32-8M (PCI)
      | Inc. Encoder
      | Slot: [1, 13]
  Mux : Mux  Inputs=8
  enc 1 : xpcconteclib/Incremental Encoder/CNT32-8M(PCI)   Channel=1  OperationMode=2-phase Input Synchronous Clear Multiply by 4  DigitalFilter=No filtering  PulseInput=TTL level input  Direction=Up in the clockwise direction/Down in the counterclockwise direction  InitialValue=counter_offset_init  LoadInitialValue=on  SampleTime=dt  PciSlot=[1,13]  StartMethod=Model Start  StopMethod=Model Terminate  ZeroClearRising=off  ZeroClearFalling=off  ZeroClearMatch0=off  ZeroClearMatch1=off  PresetRising=on  PresetFalling=off  PresetMatch0=off  PresetMatch1=off  PresetValue=0  Match0Value=0  Match1Value=0  OutputSignalMatch0=off  OutputSignalMatch1=off  OutputSignalAbnormal=off  OutputSignalDigitalFilter=off  OutputSignalAlarm=off  OneShotDuration=10 microseconds  IndexEnable=Disable  IndexLogic=Positive (Active High)  EnableDigitalInput=off  EnableDigitalOutput=off  DigitalOutputInitialValue=None  DigitalOutputFinalValue=None
  enc 2 : xpcconteclib/Incremental Encoder/CNT32-8M(PCI)   Channel=2  OperationMode=2-phase Input Synchronous Clear Multiply by 4  DigitalFilter=No filtering  PulseInput=TTL level input  Direction=Up in the clockwise direction/Down in the counterclockwise direction  InitialValue=counter_offset_init  LoadInitialValue=on  SampleTime=dt  PciSlot=[1,13]  StartMethod=Model Start  StopMethod=Model Terminate  ZeroClearRising=off  ZeroClearFalling=off  ZeroClearMatch0=off  ZeroClearMatch1=off  PresetRising=off  PresetFalling=off  PresetMatch0=off  PresetMatch1=off  PresetValue=0  Match0Value=0  Match1Value=0  OutputSignalMatch0=off  OutputSignalMatch1=off  OutputSignalAbnormal=off  OutputSignalDigitalFilter=off  OutputSignalAlarm=off  OneShotDuration=10 microseconds  IndexEnable=Disable  IndexLogic=Positive (Active High)  EnableDigitalInput=off  EnableDigitalOutput=off  DigitalOutputInitialValue=None  DigitalOutputFinalValue=None
  enc 3 : xpcconteclib/Incremental Encoder/CNT32-8M(PCI)   Channel=3  OperationMode=2-phase Input Synchronous Clear Multiply by 4  DigitalFilter=No filtering  PulseInput=TTL level input  Direction=Down in the clockwise direction/Up in the counterclockwise direction  InitialValue=counter_offset_init  LoadInitialValue=on  SampleTime=dt  PciSlot=[1,13]  StartMethod=Model Start  StopMethod=Model Terminate  ZeroClearRising=off  ZeroClearFalling=off  ZeroClearMatch0=off  ZeroClearMatch1=off  PresetRising=off  PresetFalling=off  PresetMatch0=off  PresetMatch1=off  PresetValue=0  Match0Value=0  Match1Value=0  OutputSignalMatch0=off  OutputSignalMatch1=off  OutputSignalAbnormal=off  OutputSignalDigitalFilter=off  OutputSignalAlarm=off  OneShotDuration=10 microseconds  IndexEnable=Disable  IndexLogic=Positive (Active High)  EnableDigitalInput=off  EnableDigitalOutput=off  DigitalOutputInitialValue=None  DigitalOutputFinalValue=None
  enc 4 : xpcconteclib/Incremental Encoder/CNT32-8M(PCI)   Channel=4  OperationMode=2-phase Input Synchronous Clear Multiply by 4  DigitalFilter=No filtering  PulseInput=TTL level input  Direction=Down in the clockwise direction/Up in the counterclockwise direction  InitialValue=counter_offset_init  LoadInitialValue=on  SampleTime=dt  PciSlot=[1,13]  StartMethod=Model Start  StopMethod=Model Terminate  ZeroClearRising=off  ZeroClearFalling=off  ZeroClearMatch0=off  ZeroClearMatch1=off  PresetRising=off  PresetFalling=off  PresetMatch0=off  PresetMatch1=off  PresetValue=0  Match0Value=0  Match1Value=0  OutputSignalMatch0=off  OutputSignalMatch1=off  OutputSignalAbnormal=off  OutputSignalDigitalFilter=off  OutputSignalAlarm=off  OneShotDuration=10 microseconds  IndexEnable=Disable  IndexLogic=Positive (Active High)  EnableDigitalInput=off  EnableDigitalOutput=off  DigitalOutputInitialValue=None  DigitalOutputFinalValue=None
  enc 5 : xpcconteclib/Incremental Encoder/CNT32-8M(PCI)   Channel=5  OperationMode=2-phase Input Synchronous Clear Multiply by 4  DigitalFilter=No filtering  PulseInput=TTL level input  Direction=Up in the clockwise direction/Down in the counterclockwise direction  InitialValue=counter_offset_init  LoadInitialValue=on  SampleTime=dt  PciSlot=[1,13]  StartMethod=Model Start  StopMethod=Model Terminate  ZeroClearRising=off  ZeroClearFalling=off  ZeroClearMatch0=off  ZeroClearMatch1=off  PresetRising=off  PresetFalling=off  PresetMatch0=off  PresetMatch1=off  PresetValue=0  Match0Value=0  Match1Value=0  OutputSignalMatch0=off  OutputSignalMatch1=off  OutputSignalAbnormal=off  OutputSignalDigitalFilter=off  OutputSignalAlarm=off  OneShotDuration=10 microseconds  IndexEnable=Disable  IndexLogic=Positive (Active High)  EnableDigitalInput=off  EnableDigitalOutput=off  DigitalOutputInitialValue=None  DigitalOutputFinalValue=None
  enc 6 : xpcconteclib/Incremental Encoder/CNT32-8M(PCI)   Channel=6  OperationMode=2-phase Input Synchronous Clear Multiply by 4  DigitalFilter=No filtering  PulseInput=TTL level input  Direction=Up in the clockwise direction/Down in the counterclockwise direction  InitialValue=counter_offset_init  LoadInitialValue=on  SampleTime=dt  PciSlot=[1,13]  StartMethod=Model Start  StopMethod=Model Terminate  ZeroClearRising=off  ZeroClearFalling=off  ZeroClearMatch0=off  ZeroClearMatch1=off  PresetRising=off  PresetFalling=off  PresetMatch0=off  PresetMatch1=off  PresetValue=0  Match0Value=0  Match1Value=0  OutputSignalMatch0=off  OutputSignalMatch1=off  OutputSignalAbnormal=off  OutputSignalDigitalFilter=off  OutputSignalAlarm=off  OneShotDuration=10 microseconds  IndexEnable=Disable  IndexLogic=Positive (Active High)  EnableDigitalInput=off  EnableDigitalOutput=off  DigitalOutputInitialValue=None  DigitalOutputFinalValue=None
  enc 7 : xpcconteclib/Incremental Encoder/CNT32-8M(PCI)   Channel=7  OperationMode=2-phase Input Synchronous Clear Multiply by 4  DigitalFilter=No filtering  PulseInput=TTL level input  Direction=Down in the clockwise direction/Up in the counterclockwise direction  InitialValue=counter_offset_init  LoadInitialValue=on  SampleTime=dt  PciSlot=[1,13]  StartMethod=Model Start  StopMethod=Model Terminate  ZeroClearRising=off  ZeroClearFalling=off  ZeroClearMatch0=off  ZeroClearMatch1=off  PresetRising=off  PresetFalling=off  PresetMatch0=off  PresetMatch1=off  PresetValue=0  Match0Value=0  Match1Value=0  OutputSignalMatch0=off  OutputSignalMatch1=off  OutputSignalAbnormal=off  OutputSignalDigitalFilter=off  OutputSignalAlarm=off  OneShotDuration=10 microseconds  IndexEnable=Disable  IndexLogic=Positive (Active High)  EnableDigitalInput=off  EnableDigitalOutput=off  DigitalOutputInitialValue=None  DigitalOutputFinalValue=None
  enc 8 : xpcconteclib/Incremental Encoder/CNT32-8M(PCI)   Channel=8  OperationMode=2-phase Input Synchronous Clear Multiply by 4  DigitalFilter=No filtering  PulseInput=TTL level input  Direction=Down in the clockwise direction/Up in the counterclockwise direction  InitialValue=counter_offset_init  LoadInitialValue=on  SampleTime=dt  PciSlot=[1,13]  StartMethod=Model Start  StopMethod=Model Terminate  ZeroClearRising=off  ZeroClearFalling=off  ZeroClearMatch0=off  ZeroClearMatch1=off  PresetRising=off  PresetFalling=off  PresetMatch0=off  PresetMatch1=off  PresetValue=0  Match0Value=0  Match1Value=0  OutputSignalMatch0=off  OutputSignalMatch1=off  OutputSignalAbnormal=off  OutputSignalDigitalFilter=off  OutputSignalAlarm=off  OneShotDuration=10 microseconds  IndexEnable=Disable  IndexLogic=Positive (Active High)  EnableDigitalInput=off  EnableDigitalOutput=off  DigitalOutputInitialValue=None  DigitalOutputFinalValue=None
  Out1 : Outport
  wires:
  Mux/1 -> Out1/1
  enc 1/1 -> Mux/1
  enc 2/1 -> Mux/2
  enc 3/1 -> Mux/3
  enc 4/1 -> Mux/4
  enc 5/1 -> Mux/5
  enc 6/1 -> Mux/6
  enc 7/1 -> Mux/7
  enc 8/1 -> Mux/8

== system irep_force_control_m15/In-Vivo System/CONTEC CARDS/Level 2 ==
  note: Contec
      | CNT32-8M (PCI)
      | Inc. Encoder
      | Slot: [2, 8]
  Mux : Mux  Inputs=8
  enc 1 : xpcconteclib/Incremental Encoder/CNT32-8M(PCI)   Channel=1  OperationMode=2-phase Input Synchronous Clear Multiply by 4  DigitalFilter=No filtering  PulseInput=TTL level input  Direction=Down in the clockwise direction/Up in the counterclockwise direction  InitialValue=counter_offset_init  LoadInitialValue=on  SampleTime=dt  PciSlot=[2,8]  StartMethod=Model Start  StopMethod=Model Terminate  ZeroClearRising=off  ZeroClearFalling=off  ZeroClearMatch0=off  ZeroClearMatch1=off  PresetRising=on  PresetFalling=off  PresetMatch0=off  PresetMatch1=off  PresetValue=0  Match0Value=0  Match1Value=0  OutputSignalMatch0=off  OutputSignalMatch1=off  OutputSignalAbnormal=off  OutputSignalDigitalFilter=off  OutputSignalAlarm=off  OneShotDuration=10 microseconds  IndexEnable=Disable  IndexLogic=Positive (Active High)  EnableDigitalInput=off  EnableDigitalOutput=off  DigitalOutputInitialValue=None  DigitalOutputFinalValue=None
  enc 2 : xpcconteclib/Incremental Encoder/CNT32-8M(PCI)   Channel=2  OperationMode=2-phase Input Synchronous Clear Multiply by 4  DigitalFilter=No filtering  PulseInput=TTL level input  Direction=Up in the clockwise direction/Down in the counterclockwise direction  InitialValue=counter_offset_init  LoadInitialValue=on  SampleTime=dt  PciSlot=[2,8]  StartMethod=Model Start  StopMethod=Model Terminate  ZeroClearRising=off  ZeroClearFalling=off  ZeroClearMatch0=off  ZeroClearMatch1=off  PresetRising=off  PresetFalling=off  PresetMatch0=off  PresetMatch1=off  PresetValue=0  Match0Value=0  Match1Value=0  OutputSignalMatch0=off  OutputSignalMatch1=off  OutputSignalAbnormal=off  OutputSignalDigitalFilter=off  OutputSignalAlarm=off  OneShotDuration=10 microseconds  IndexEnable=Disable  IndexLogic=Positive (Active High)  EnableDigitalInput=off  EnableDigitalOutput=off  DigitalOutputInitialValue=None  DigitalOutputFinalValue=None
  enc 3 : xpcconteclib/Incremental Encoder/CNT32-8M(PCI)   Channel=3  OperationMode=2-phase Input Synchronous Clear Multiply by 4  DigitalFilter=No filtering  PulseInput=TTL level input  Direction=Up in the clockwise direction/Down in the counterclockwise direction  InitialValue=counter_offset_init  LoadInitialValue=on  SampleTime=dt  PciSlot=[2,8]  StartMethod=Model Start  StopMethod=Model Terminate  ZeroClearRising=off  ZeroClearFalling=off  ZeroClearMatch0=off  ZeroClearMatch1=off  PresetRising=off  PresetFalling=off  PresetMatch0=off  PresetMatch1=off  PresetValue=0  Match0Value=0  Match1Value=0  OutputSignalMatch0=off  OutputSignalMatch1=off  OutputSignalAbnormal=off  OutputSignalDigitalFilter=off  OutputSignalAlarm=off  OneShotDuration=10 microseconds  IndexEnable=Disable  IndexLogic=Positive (Active High)  EnableDigitalInput=off  EnableDigitalOutput=off  DigitalOutputInitialValue=None  DigitalOutputFinalValue=None
  enc 4 : xpcconteclib/Incremental Encoder/CNT32-8M(PCI)   Channel=4  OperationMode=2-phase Input Synchronous Clear Multiply by 4  DigitalFilter=No filtering  PulseInput=TTL level input  Direction=Up in the clockwise direction/Down in the counterclockwise direction  InitialValue=counter_offset_init  LoadInitialValue=on  SampleTime=dt  PciSlot=[2,8]  StartMethod=Model Start  StopMethod=Model Terminate  ZeroClearRising=off  ZeroClearFalling=off  ZeroClearMatch0=off  ZeroClearMatch1=off  PresetRising=off  PresetFalling=off  PresetMatch0=off  PresetMatch1=off  PresetValue=0  Match0Value=0  Match1Value=0  OutputSignalMatch0=off  OutputSignalMatch1=off  OutputSignalAbnormal=off  OutputSignalDigitalFilter=off  OutputSignalAlarm=off  OneShotDuration=10 microseconds  IndexEnable=Disable  IndexLogic=Positive (Active High)  EnableDigitalInput=off  EnableDigitalOutput=off  DigitalOutputInitialValue=None  DigitalOutputFinalValue=None
  enc 5 : xpcconteclib/Incremental Encoder/CNT32-8M(PCI)   Channel=5  OperationMode=2-phase Input Synchronous Clear Multiply by 4  DigitalFilter=No filtering  PulseInput=TTL level input  Direction=Up in the clockwise direction/Down in the counterclockwise direction  InitialValue=counter_offset_init  LoadInitialValue=on  SampleTime=dt  PciSlot=[2,8]  StartMethod=Model Start  StopMethod=Model Terminate  ZeroClearRising=off  ZeroClearFalling=off  ZeroClearMatch0=off  ZeroClearMatch1=off  PresetRising=off  PresetFalling=off  PresetMatch0=off  PresetMatch1=off  PresetValue=0  Match0Value=0  Match1Value=0  OutputSignalMatch0=off  OutputSignalMatch1=off  OutputSignalAbnormal=off  OutputSignalDigitalFilter=off  OutputSignalAlarm=off  OneShotDuration=10 microseconds  IndexEnable=Disable  IndexLogic=Positive (Active High)  EnableDigitalInput=off  EnableDigitalOutput=off  DigitalOutputInitialValue=None  DigitalOutputFinalValue=None
  enc 6 : xpcconteclib/Incremental Encoder/CNT32-8M(PCI)   Channel=6  OperationMode=2-phase Input Synchronous Clear Multiply by 4  DigitalFilter=No filtering  PulseInput=TTL level input  Direction=Down in the clockwise direction/Up in the counterclockwise direction  InitialValue=counter_offset_init  LoadInitialValue=on  SampleTime=dt  PciSlot=[2,8]  StartMethod=Model Start  StopMethod=Model Terminate  ZeroClearRising=off  ZeroClearFalling=off  ZeroClearMatch0=off  ZeroClearMatch1=off  PresetRising=off  PresetFalling=off  PresetMatch0=off  PresetMatch1=off  PresetValue=0  Match0Value=0  Match1Value=0  OutputSignalMatch0=off  OutputSignalMatch1=off  OutputSignalAbnormal=off  OutputSignalDigitalFilter=off  OutputSignalAlarm=off  OneShotDuration=10 microseconds  IndexEnable=Disable  IndexLogic=Positive (Active High)  EnableDigitalInput=off  EnableDigitalOutput=off  DigitalOutputInitialValue=None  DigitalOutputFinalValue=None
  enc 7 : xpcconteclib/Incremental Encoder/CNT32-8M(PCI)   Channel=7  OperationMode=2-phase Input Synchronous Clear Multiply by 4  DigitalFilter=No filtering  PulseInput=TTL level input  Direction=Down in the clockwise direction/Up in the counterclockwise direction  InitialValue=counter_offset_init  LoadInitialValue=on  SampleTime=dt  PciSlot=[2,8]  StartMethod=Model Start  StopMethod=Model Terminate  ZeroClearRising=off  ZeroClearFalling=off  ZeroClearMatch0=off  ZeroClearMatch1=off  PresetRising=off  PresetFalling=off  PresetMatch0=off  PresetMatch1=off  PresetValue=0  Match0Value=0  Match1Value=0  OutputSignalMatch0=off  OutputSignalMatch1=off  OutputSignalAbnormal=off  OutputSignalDigitalFilter=off  OutputSignalAlarm=off  OneShotDuration=10 microseconds  IndexEnable=Disable  IndexLogic=Positive (Active High)  EnableDigitalInput=off  EnableDigitalOutput=off  DigitalOutputInitialValue=None  DigitalOutputFinalValue=None
  enc 8 : xpcconteclib/Incremental Encoder/CNT32-8M(PCI)   Channel=8  OperationMode=2-phase Input Synchronous Clear Multiply by 4  DigitalFilter=No filtering  PulseInput=TTL level input  Direction=Down in the clockwise direction/Up in the counterclockwise direction  InitialValue=counter_offset_init  LoadInitialValue=on  SampleTime=dt  PciSlot=[2,8]  StartMethod=Model Start  StopMethod=Model Terminate  ZeroClearRising=off  ZeroClearFalling=off  ZeroClearMatch0=off  ZeroClearMatch1=off  PresetRising=off  PresetFalling=off  PresetMatch0=off  PresetMatch1=off  PresetValue=0  Match0Value=0  Match1Value=0  OutputSignalMatch0=off  OutputSignalMatch1=off  OutputSignalAbnormal=off  OutputSignalDigitalFilter=off  OutputSignalAlarm=off  OneShotDuration=10 microseconds  IndexEnable=Disable  IndexLogic=Positive (Active High)  EnableDigitalInput=off  EnableDigitalOutput=off  DigitalOutputInitialValue=None  DigitalOutputFinalValue=None
  Out1 : Outport
  wires:
  Mux/1 -> Out1/1
  enc 5/1 -> Mux/5
  enc 1/1 -> Mux/1
  enc 3/1 -> Mux/3
  enc 7/1 -> Mux/7
  enc 6/1 -> Mux/6
  enc 4/1 -> Mux/4
  enc 2/1 -> Mux/2
  enc 8/1 -> Mux/8
